simulink model "sgMdl_ModbusTCP_1CLI3SRV"  (R2024b)
settings: Solver=FixedStepAuto  StartTime=0.0  StopTime=inf  RelTol=1e-3  EnableMultiTasking=on
libraries: speedgoatlib_mbtcp x27, slrealtimeutilitieslib x20
Description:
  | Native Modbus TCP Multi-Node Loopback
settings Model: sg_rtwmakecfg_data=_sg_IO75X_v1_2_0__sg_netxLib_MSVC140_  ModifiedByFormat=Speedgoat  SimulationMode=external  ExtModeTrigDuration=100000  Creator=Speedgoat  LastModifiedBy=Speedgoat
settings SolverCC: ConcurrentTasks=on  AlgebraicLoopSolver=TrustRegion  PositivePriorityOrder=on  AutoInsertRateTranBlk=on  InsertRTBMode=Never (minimum delay)
settings DataIOCC: LimitDataPoints=on  SaveFormat=StructureWithTime  ReturnWorkspaceOutputs=off
settings OptimizationCC: BlockReduction=off  BooleanDataType=off  OptimizeBlockIOStorage=off  BufferReuse=off  GlobalBufferReuse=off  ExpressionFolding=off  LocalBlockOutputs=off  OptimizeDataStoreBuffers=off  BusAssignmentInplaceUpdate=off
settings DebuggingCC: SaveWithParameterizedLinksMsg=none  UnderspecifiedInitializationDetection=Classic  MergeDetectMultiDrivingBlocksExec=none  SignalResolutionControl=TryResolveAllWithWarning  InheritedTsInSrcMsg=none  TasksWithSamePriorityMsg=none  ParameterOverflowMsg=warning  UnconnectedInputMsg=warning  UnconnectedOutputMsg=warning  UnconnectedLineMsg=warning  SFUnexpectedBacktrackingDiag=warning  SFNoUnconditionalDefaultTransitionDiag=warning  SFExecutionAtInitializationDiag=none  ArithmeticOperatorsInVariantConditions=warning
settings HardwareCC: ProdBitPerLong=64  ProdLongLongMode=on  ProdHWDeviceType=Intel->x86-64 (Linux 64)  TargetBitPerPointer=64  TargetBitPerSizeT=64  TargetBitPerPtrDiffT=64  TargetLongLongMode=on  TargetIntDivRoundTo=Zero  TargetEndianess=LittleEndian  TargetWordSize=64  TargetHWDeviceType=MATLAB Host
settings ModelReferenceCC: EnableRefExpFcnMdlSchedulingChecks=on  PropagateSignalLabelsOutOfModel=off
settings SFSimCC: SimUseLocalCustomCode=off  CustomCodeUndefinedFunction=UseInterfaceOnly
settings RTWCC: Description=Speedgoat Real-Time Target Machine  SystemTargetFile=speedgoat.tlc  TemplateMakefile=slrealtime_default_tmf  RetainRTWFile=on  RTWUseLocalCustomCode=off  Toolchain=Simulink Real-Time Toolchain  BuildConfiguration=Faster Runs  TargetLang=C++  GPUComputeCapability=3.5  DLArmComputeVersion=19.05
settings CodeAppCC: StateflowObjectComments=on
settings SimulinkRealTimeTargetCC: SubcomponentCodeInterfacePackaging=Reusable function  InstructionSetFMA=off  LogToMDFFile=off  SLRTFileLogMaxRuns=10  UseGCCFastMath=on
settings ConfigComp: CovMetricSettings=dw  CovSaveCumulativeToWorkspaceVar=on  CovSaveSingleToWorkspaceVar=on  CovExternalEMLEnable=off  CovBoundaryAbsTol=1.0e-5

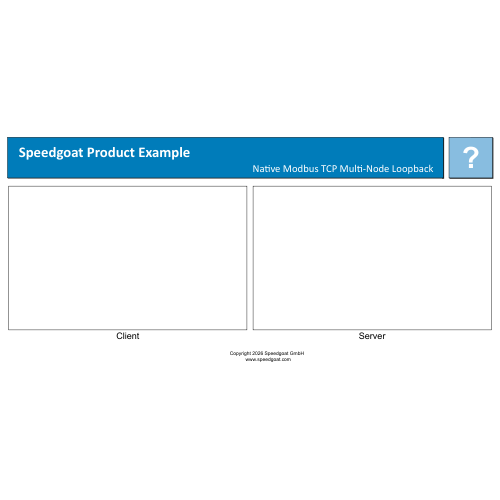
[thumbnail: Simulink's stored preview of the top-level diagram]
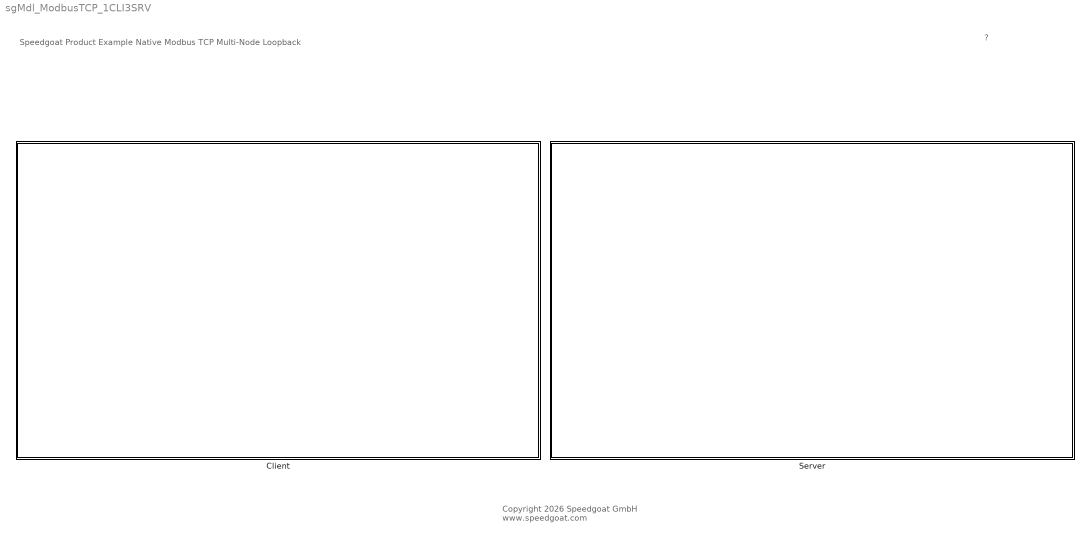
== system sgMdl_ModbusTCP_1CLI3SRV ==
  note: Speedgoat Product Example
      | Native Modbus TCP Multi-Node Loopback
  note: ?
  note: Copyright 2026 Speedgoat GmbH
      |  www.speedgoat.com
  Client : Subsystem
  Server : Subsystem

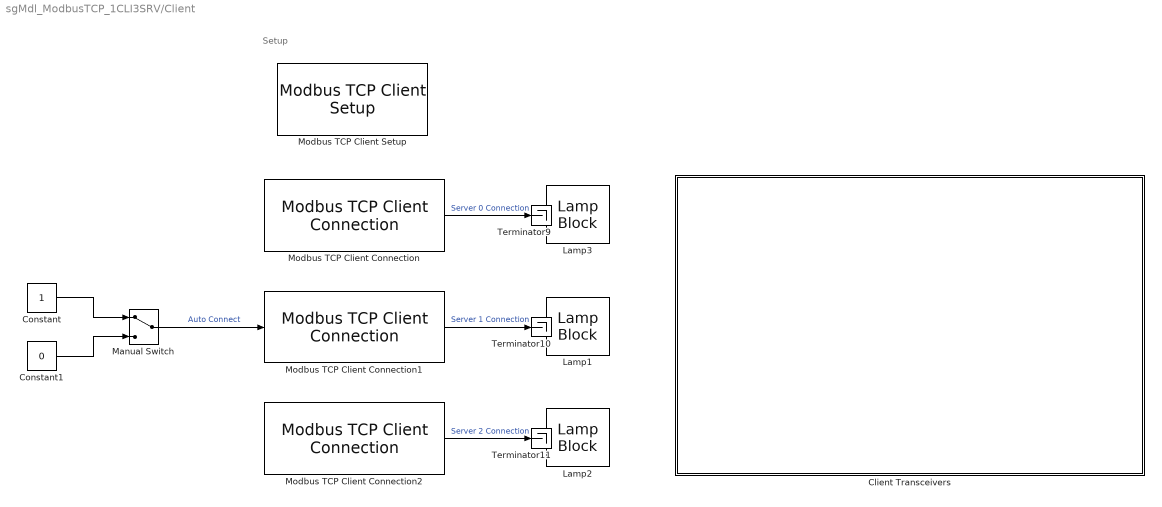
== system sgMdl_ModbusTCP_1CLI3SRV/Client ==
  note: Setup
  Client Transceivers : Subsystem
  Constant : Constant  OutDataTypeStr=boolean
  Constant1 : Constant  Value=0  OutDataTypeStr=boolean
  Lamp1 : LampBlock  LabelPosition=Bottom
  Lamp2 : LampBlock  LabelPosition=Bottom
  Lamp3 : LampBlock  LabelPosition=Bottom
  Manual Switch : ManualSwitch
  Modbus TCP Client Connection : speedgoatlib_mbtcp/Client/Modbus TCP Client Connection  ClientID=10  ConnectionID=0  remoteipAddrStr=IP_Server_00  remoteTCPPort=502  DataSwap=off  parConcurrence=on  AutoConnect=on  SampleTime=-1
      settings: SourceProductName=Simulink Real-Time: Speedgoat I/O Blockset
      settings: AttributesFormatString=|
      | Remote IP: %<remoteipAddrStr>
      | Remote TCP Port: %<remoteTCPPort> | Data Swap: %<DataSwap>
  Modbus TCP Client Connection1 : speedgoatlib_mbtcp/Client/Modbus TCP Client Connection  ClientID=10  ConnectionID=1  remoteipAddrStr=IP_Server_01  remoteTCPPort=502  DataSwap=off  parConcurrence=on  AutoConnect=off  SampleTime=-1
      settings: SourceProductName=Simulink Real-Time: Speedgoat I/O Blockset
      settings: AttributesFormatString=|
      | Remote IP: %<remoteipAddrStr>
      | Remote TCP Port: %<remoteTCPPort> | Data Swap: %<DataSwap>
  Modbus TCP Client Connection2 : speedgoatlib_mbtcp/Client/Modbus TCP Client Connection  ClientID=10  ConnectionID=2  remoteipAddrStr=IP_Server_02  remoteTCPPort=502  DataSwap=off  parConcurrence=on  AutoConnect=on  SampleTime=-1
      settings: SourceProductName=Simulink Real-Time: Speedgoat I/O Blockset
      settings: AttributesFormatString=|
      | Remote IP: %<remoteipAddrStr>
      | Remote TCP Port: %<remoteTCPPort> | Data Swap: %<DataSwap>
  Modbus TCP Client Setup : speedgoatlib_mbtcp/Client/Modbus TCP Client Setup  ClientID=10  IpAddrStr=IP_Client_00  SampleTime=-1
      settings: AttributesFormatString=Local IP: %<IpAddrStr>  SourceProductName=Simulink Real-Time: Speedgoat I/O Blockset
  Terminator10 : Terminator
  Terminator11 : Terminator
  Terminator9 : Terminator
  wires:
  Constant1/1 -> Manual Switch/2
  Constant/1 -> Manual Switch/1
  Modbus TCP Client Connection1/1 -> Terminator10/1  "Server 1 Connection"
  Modbus TCP Client Connection2/1 -> Terminator11/1  "Server 2 Connection"
  Manual Switch/1 -> Modbus TCP Client Connection1/1  "Auto Connect"
  Modbus TCP Client Connection/1 -> Terminator9/1  "Server 0 Connection"

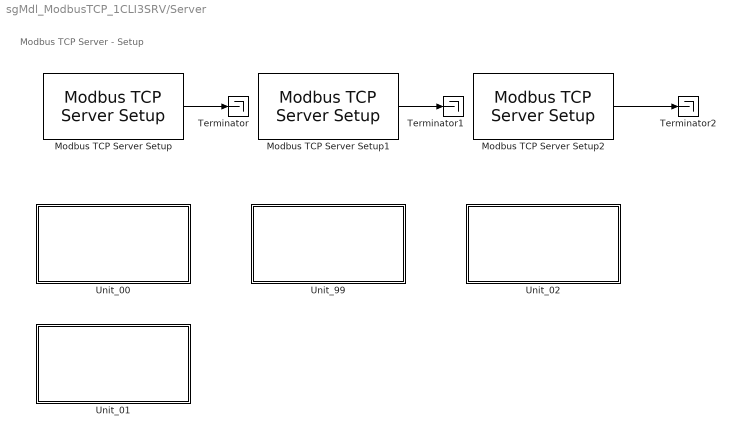
== system sgMdl_ModbusTCP_1CLI3SRV/Server ==
  note: Modbus TCP Server - Setup
  Modbus TCP Server Setup : speedgoatlib_mbtcp/Server/Modbus TCP Server Setup  ServerID=0  IpAddrStr=IP_Server_00  TcpPort=502  Units=[0,1]  TableDim=[10,10,10,10;255,255,255,255]  RespDelay=0  ByteSwap=off  KeepAlive=1  SampleTime=-1
      settings: SourceProductName=Simulink Real-Time: Speedgoat I/O Blockset
      settings: AttributesFormatString=|
      | Local IP: %<IpAddrStr>
      | Local TCP Port: %<TCPPort> | Units: %<Units>
  Modbus TCP Server Setup1 : speedgoatlib_mbtcp/Server/Modbus TCP Server Setup  ServerID=1  IpAddrStr=IP_Server_01  TcpPort=502  Units=[99]  TableDim=[64,64,64,64]  RespDelay=0  ByteSwap=off  KeepAlive=0  SampleTime=-1
      settings: SourceProductName=Simulink Real-Time: Speedgoat I/O Blockset
      settings: AttributesFormatString=|
      | Local IP: %<IpAddrStr>
      | Local TCP Port: %<TCPPort> | Units: %<Units>
  Modbus TCP Server Setup2 : speedgoatlib_mbtcp/Server/Modbus TCP Server Setup  ServerID=2  IpAddrStr=IP_Server_02  TcpPort=502  Units=[2]  TableDim=[64,64,64,64]  RespDelay=0  ByteSwap=off  KeepAlive=0  SampleTime=-1
      settings: SourceProductName=Simulink Real-Time: Speedgoat I/O Blockset
      settings: AttributesFormatString=|
      | Local IP: %<IpAddrStr>
      | Local TCP Port: %<TCPPort> | Units: %<Units>
  Terminator : Terminator
  Terminator1 : Terminator
  Terminator2 : Terminator
  Unit_00 : Subsystem
  Unit_01 : Subsystem
  Unit_02 : Subsystem
  Unit_99 : Subsystem
  wires:
  Modbus TCP Server Setup2/1 -> Terminator2/1
  Modbus TCP Server Setup1/1 -> Terminator1/1
  Modbus TCP Server Setup/1 -> Terminator/1

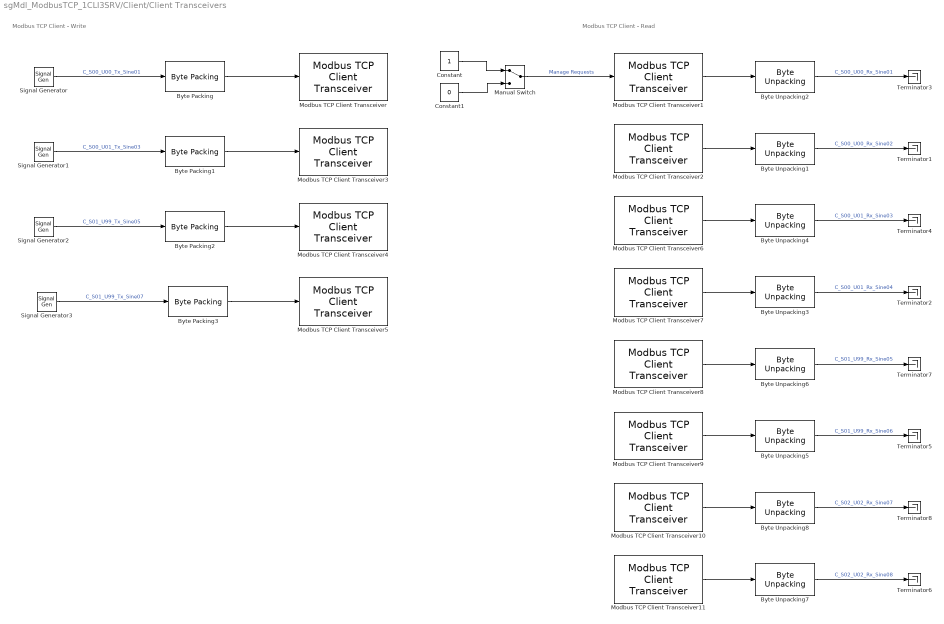
== system sgMdl_ModbusTCP_1CLI3SRV/Client/Client Transceivers ==
  note: Modbus TCP Client - Write
  note: Modbus TCP Client - Read
  Byte Packing{,1..3} (4 alike) : slrealtimeutilitieslib/Byte Packing  MaskPackedDataType=uint16  MaskUnpackedDataTypes={'double'}  MaskAlignment=1
  Byte Unpacking{1..8} (8 alike) : slrealtimeutilitieslib/Byte Unpacking  MaskUnpackedDataTypes={'double'}  MaskUnpackedDataSizes={[1]}  MaskAlignment=1
  Constant : Constant  OutDataTypeStr=boolean
  Constant1 : Constant  Value=0  OutDataTypeStr=boolean
  Manual Switch : ManualSwitch
  Modbus TCP Client Transceiver : speedgoatlib_mbtcp/Client/Modbus TCP Client Transceiver  ClientID=10  ConnectionID=0  remoteUnitID=0  FunctionCode=FC16 (Write Multiple Holding Registers)  DataIndex=0  DataQuantity=4  PollIntervall=50  EnaSend=off  SampleTime=-1  UpdateChange=off
      settings: SourceProductName=Simulink Real-Time: Speedgoat I/O Blockset
      settings: AttributesFormatString=|
      | %<FunctionCode>
      | Server Unit: %<remoteUnitID> | Address Index: %<DataIndex> | Quantity: %<DataQuantity>
  Modbus TCP Client Transceiver1 : speedgoatlib_mbtcp/Client/Modbus TCP Client Transceiver  ClientID=10  ConnectionID=0  remoteUnitID=0  FunctionCode=FC3 (Read Multiple Holding Registers)  DataIndex=0  DataQuantity=4  PollIntervall=50  EnaSend=on  SampleTime=-1  UpdateChange=off
      settings: SourceProductName=Simulink Real-Time: Speedgoat I/O Blockset
      settings: AttributesFormatString=|
      | %<FunctionCode>
      | Server Unit: %<remoteUnitID> | Address Index: %<DataIndex> | Quantity: %<DataQuantity>
  Modbus TCP Client Transceiver10 : speedgoatlib_mbtcp/Client/Modbus TCP Client Transceiver  ClientID=10  ConnectionID=2  remoteUnitID=2  FunctionCode=FC3 (Read Multiple Holding Registers)  DataIndex=0  DataQuantity=4  PollIntervall=50  EnaSend=off  SampleTime=-1  UpdateChange=off
      settings: SourceProductName=Simulink Real-Time: Speedgoat I/O Blockset
      settings: AttributesFormatString=|
      | %<FunctionCode>
      | Server Unit: %<remoteUnitID> | Address Index: %<DataIndex> | Quantity: %<DataQuantity>
  Modbus TCP Client Transceiver11 : speedgoatlib_mbtcp/Client/Modbus TCP Client Transceiver  ClientID=10  ConnectionID=2  remoteUnitID=2  FunctionCode=FC4 (Read Multiple Input Registers)  DataIndex=0  DataQuantity=4  PollIntervall=50  EnaSend=off  SampleTime=-1  UpdateChange=off
      settings: SourceProductName=Simulink Real-Time: Speedgoat I/O Blockset
      settings: AttributesFormatString=|
      | %<FunctionCode>
      | Server Unit: %<remoteUnitID> | Address Index: %<DataIndex> | Quantity: %<DataQuantity>
  Modbus TCP Client Transceiver2 : speedgoatlib_mbtcp/Client/Modbus TCP Client Transceiver  ClientID=10  ConnectionID=0  remoteUnitID=0  FunctionCode=FC4 (Read Multiple Input Registers)  DataIndex=0  DataQuantity=4  PollIntervall=50  EnaSend=off  SampleTime=-1  UpdateChange=off
      settings: SourceProductName=Simulink Real-Time: Speedgoat I/O Blockset
      settings: AttributesFormatString=|
      | %<FunctionCode>
      | Server Unit: %<remoteUnitID> | Address Index: %<DataIndex> | Quantity: %<DataQuantity>
  Modbus TCP Client Transceiver3 : speedgoatlib_mbtcp/Client/Modbus TCP Client Transceiver  ClientID=10  ConnectionID=0  remoteUnitID=1  FunctionCode=FC16 (Write Multiple Holding Registers)  DataIndex=0  DataQuantity=4  PollIntervall=50  EnaSend=off  SampleTime=-1  UpdateChange=off
      settings: SourceProductName=Simulink Real-Time: Speedgoat I/O Blockset
      settings: AttributesFormatString=|
      | %<FunctionCode>
      | Server Unit: %<remoteUnitID> | Address Index: %<DataIndex> | Quantity: %<DataQuantity>
  Modbus TCP Client Transceiver4 : speedgoatlib_mbtcp/Client/Modbus TCP Client Transceiver  ClientID=10  ConnectionID=1  remoteUnitID=99  FunctionCode=FC16 (Write Multiple Holding Registers)  DataIndex=0  DataQuantity=4  PollIntervall=50  EnaSend=off  SampleTime=-1  UpdateChange=off
      settings: SourceProductName=Simulink Real-Time: Speedgoat I/O Blockset
      settings: AttributesFormatString=|
      | %<FunctionCode>
      | Server Unit: %<remoteUnitID> | Address Index: %<DataIndex> | Quantity: %<DataQuantity>
  Modbus TCP Client Transceiver5 : speedgoatlib_mbtcp/Client/Modbus TCP Client Transceiver  ClientID=10  ConnectionID=2  remoteUnitID=2  FunctionCode=FC16 (Write Multiple Holding Registers)  DataIndex=0  DataQuantity=4  PollIntervall=50  EnaSend=off  SampleTime=-1  UpdateChange=off
      settings: SourceProductName=Simulink Real-Time: Speedgoat I/O Blockset
      settings: AttributesFormatString=|
      | %<FunctionCode>
      | Server Unit: %<remoteUnitID> | Address Index: %<DataIndex> | Quantity: %<DataQuantity>
  Modbus TCP Client Transceiver6 : speedgoatlib_mbtcp/Client/Modbus TCP Client Transceiver  ClientID=10  ConnectionID=0  remoteUnitID=1  FunctionCode=FC3 (Read Multiple Holding Registers)  DataIndex=0  DataQuantity=4  PollIntervall=50  EnaSend=off  SampleTime=-1  UpdateChange=off
      settings: SourceProductName=Simulink Real-Time: Speedgoat I/O Blockset
      settings: AttributesFormatString=|
      | %<FunctionCode>
      | Server Unit: %<remoteUnitID> | Address Index: %<DataIndex> | Quantity: %<DataQuantity>
  Modbus TCP Client Transceiver7 : speedgoatlib_mbtcp/Client/Modbus TCP Client Transceiver  ClientID=10  ConnectionID=0  remoteUnitID=1  FunctionCode=FC4 (Read Multiple Input Registers)  DataIndex=0  DataQuantity=4  PollIntervall=50  EnaSend=off  SampleTime=-1  UpdateChange=off
      settings: SourceProductName=Simulink Real-Time: Speedgoat I/O Blockset
      settings: AttributesFormatString=|
      | %<FunctionCode>
      | Server Unit: %<remoteUnitID> | Address Index: %<DataIndex> | Quantity: %<DataQuantity>
  Modbus TCP Client Transceiver8 : speedgoatlib_mbtcp/Client/Modbus TCP Client Transceiver  ClientID=10  ConnectionID=1  remoteUnitID=99  FunctionCode=FC3 (Read Multiple Holding Registers)  DataIndex=0  DataQuantity=4  PollIntervall=50  EnaSend=off  SampleTime=-1  UpdateChange=off
      settings: SourceProductName=Simulink Real-Time: Speedgoat I/O Blockset
      settings: AttributesFormatString=|
      | %<FunctionCode>
      | Server Unit: %<remoteUnitID> | Address Index: %<DataIndex> | Quantity: %<DataQuantity>
  Modbus TCP Client Transceiver9 : speedgoatlib_mbtcp/Client/Modbus TCP Client Transceiver  ClientID=10  ConnectionID=1  remoteUnitID=99  FunctionCode=FC4 (Read Multiple Input Registers)  DataIndex=0  DataQuantity=4  PollIntervall=50  EnaSend=off  SampleTime=-1  UpdateChange=off
      settings: SourceProductName=Simulink Real-Time: Speedgoat I/O Blockset
      settings: AttributesFormatString=|
      | %<FunctionCode>
      | Server Unit: %<remoteUnitID> | Address Index: %<DataIndex> | Quantity: %<DataQuantity>
  Signal Generator : SignalGenerator  Amplitude=10  Frequency=0.1  Units=rad/sec
  Signal Generator1 : SignalGenerator  Amplitude=30  Frequency=0.3  Units=rad/sec
  Signal Generator2 : SignalGenerator  Amplitude=50  Frequency=0.5  Units=rad/sec
  Signal Generator3 : SignalGenerator  Amplitude=70  Frequency=0.7  Units=rad/sec
  Terminator{1..8} (8 alike) : Terminator
  wires:
  Modbus TCP Client Transceiver1/1 -> Byte Unpacking2/1
  Signal Generator/1 -> Byte Packing/1  "C_S00_U00_Tx_Sine01"
  Byte Unpacking1/1 -> Terminator1/1  "C_S00_U00_Rx_Sine02"
  Modbus TCP Client Transceiver2/1 -> Byte Unpacking1/1
  Byte Packing/1 -> Modbus TCP Client Transceiver/1
  Byte Unpacking2/1 -> Terminator3/1  "C_S00_U00_Rx_Sine01"
  Signal Generator1/1 -> Byte Packing1/1  "C_S00_U01_Tx_Sine03"
  Byte Packing1/1 -> Modbus TCP Client Transceiver3/1
  Byte Packing2/1 -> Modbus TCP Client Transceiver4/1
  Signal Generator2/1 -> Byte Packing2/1  "C_S01_U99_Tx_Sine05"
  Signal Generator3/1 -> Byte Packing3/1  "C_S01_U99_Tx_Sine07"
  Byte Packing3/1 -> Modbus TCP Client Transceiver5/1
  Byte Unpacking4/1 -> Terminator4/1  "C_S00_U01_Rx_Sine03"
  Modbus TCP Client Transceiver7/1 -> Byte Unpacking3/1
  Byte Unpacking3/1 -> Terminator2/1  "C_S00_U01_Rx_Sine04"
  Modbus TCP Client Transceiver6/1 -> Byte Unpacking4/1
  Modbus TCP Client Transceiver10/1 -> Byte Unpacking8/1
  Byte Unpacking7/1 -> Terminator6/1  "C_S02_U02_Rx_Sine08"
  Modbus TCP Client Transceiver11/1 -> Byte Unpacking7/1
  Byte Unpacking8/1 -> Terminator8/1  "C_S02_U02_Rx_Sine07"
  Byte Unpacking6/1 -> Terminator7/1  "C_S01_U99_Rx_Sine05"
  Modbus TCP Client Transceiver9/1 -> Byte Unpacking5/1
  Byte Unpacking5/1 -> Terminator5/1  "C_S01_U99_Rx_Sine06"
  Modbus TCP Client Transceiver8/1 -> Byte Unpacking6/1
  Manual Switch/1 -> Modbus TCP Client Transceiver1/1  "Manage Requests"
  Constant1/1 -> Manual Switch/2
  Constant/1 -> Manual Switch/1

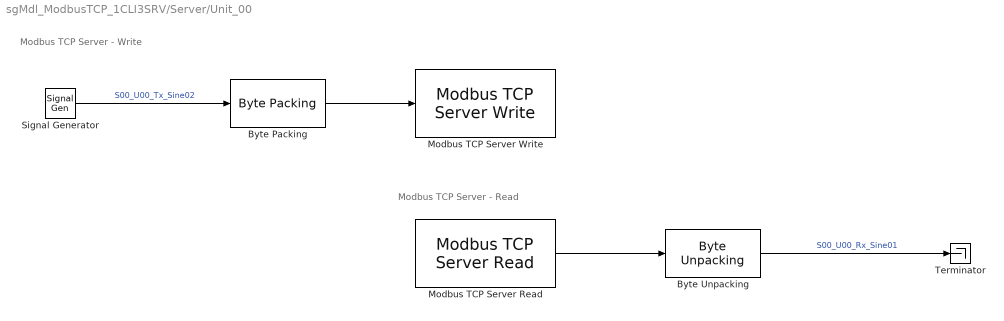
== system sgMdl_ModbusTCP_1CLI3SRV/Server/Unit_00 ==
  note: Modbus TCP Server - Write
  note: Modbus TCP Server - Read
  Byte Packing : slrealtimeutilitieslib/Byte Packing  MaskPackedDataType=uint16  MaskUnpackedDataTypes={'double'}  MaskAlignment=1
  Byte Unpacking : slrealtimeutilitieslib/Byte Unpacking  MaskUnpackedDataTypes={'double'}  MaskUnpackedDataSizes={[1]}  MaskAlignment=1
  Modbus TCP Server Read : speedgoatlib_mbtcp/Server/Modbus TCP Server Read  ServerID=0  UnitID=0  DataTable=Holding Registers  DataIndex=0  DataQuantity=4  SampleTime=-1
      settings: SourceProductName=Simulink Real-Time: Speedgoat I/O Blockset
      settings: AttributesFormatString=|
      | Data Type: %<DataTable>
      | Data Index: %<DataIndex> | Quantity: %<DataQuantity>
  Modbus TCP Server Write : speedgoatlib_mbtcp/Server/Modbus TCP Server Write  ServerID=0  UnitID=0  DataTable=Input Registers  DataIndex=0  DataQuantity=4  SampleTime=-1
      settings: SourceProductName=Simulink Real-Time: Speedgoat I/O Blockset
      settings: AttributesFormatString=|
      | Data Type: %<DataTable>
      | Data Index: %<DataIndex> | Quantity: %<DataQuantity>
  Signal Generator : SignalGenerator  Amplitude=20  Frequency=0.2  Units=rad/sec
  Terminator : Terminator
  wires:
  Modbus TCP Server Read/1 -> Byte Unpacking/1
  Byte Unpacking/1 -> Terminator/1  "S00_U00_Rx_Sine01"
  Byte Packing/1 -> Modbus TCP Server Write/1
  Signal Generator/1 -> Byte Packing/1  "S00_U00_Tx_Sine02"

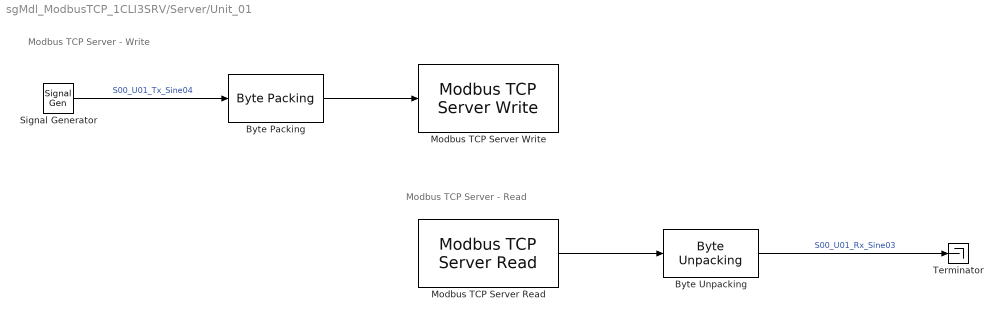
== system sgMdl_ModbusTCP_1CLI3SRV/Server/Unit_01 ==
  note: Modbus TCP Server - Read
  note: Modbus TCP Server - Write
  Byte Packing : slrealtimeutilitieslib/Byte Packing  MaskPackedDataType=uint16  MaskUnpackedDataTypes={'double'}  MaskAlignment=1
  Byte Unpacking : slrealtimeutilitieslib/Byte Unpacking  MaskUnpackedDataTypes={'double'}  MaskUnpackedDataSizes={[1]}  MaskAlignment=1
  Modbus TCP Server Read : speedgoatlib_mbtcp/Server/Modbus TCP Server Read  ServerID=0  UnitID=1  DataTable=Holding Registers  DataIndex=0  DataQuantity=4  SampleTime=-1
      settings: SourceProductName=Simulink Real-Time: Speedgoat I/O Blockset
      settings: AttributesFormatString=|
      | Data Type: %<DataTable>
      | Data Index: %<DataIndex> | Quantity: %<DataQuantity>
  Modbus TCP Server Write : speedgoatlib_mbtcp/Server/Modbus TCP Server Write  ServerID=0  UnitID=1  DataTable=Input Registers  DataIndex=0  DataQuantity=4  SampleTime=-1
      settings: SourceProductName=Simulink Real-Time: Speedgoat I/O Blockset
      settings: AttributesFormatString=|
      | Data Type: %<DataTable>
      | Data Index: %<DataIndex> | Quantity: %<DataQuantity>
  Signal Generator : SignalGenerator  Amplitude=40  Frequency=0.4  Units=rad/sec
  Terminator : Terminator
  wires:
  Signal Generator/1 -> Byte Packing/1  "S00_U01_Tx_Sine04"
  Byte Packing/1 -> Modbus TCP Server Write/1
  Byte Unpacking/1 -> Terminator/1  "S00_U01_Rx_Sine03"
  Modbus TCP Server Read/1 -> Byte Unpacking/1

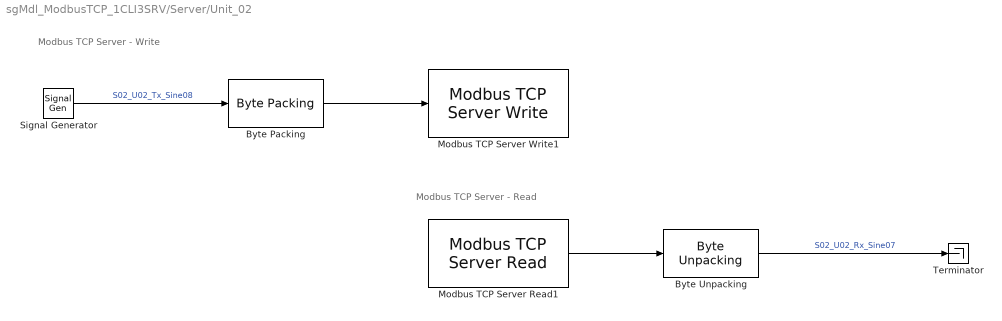
== system sgMdl_ModbusTCP_1CLI3SRV/Server/Unit_02 ==
  note: Modbus TCP Server - Read
  note: Modbus TCP Server - Write
  Byte Packing : slrealtimeutilitieslib/Byte Packing  MaskPackedDataType=uint16  MaskUnpackedDataTypes={'double'}  MaskAlignment=1
  Byte Unpacking : slrealtimeutilitieslib/Byte Unpacking  MaskUnpackedDataTypes={'double'}  MaskUnpackedDataSizes={[1]}  MaskAlignment=1
  Modbus TCP Server Read1 : speedgoatlib_mbtcp/Server/Modbus TCP Server Read  ServerID=2  UnitID=2  DataTable=Holding Registers  DataIndex=0  DataQuantity=4  SampleTime=-1
      settings: SourceProductName=Simulink Real-Time: Speedgoat I/O Blockset
      settings: AttributesFormatString=|
      | Data Type: %<DataTable>
      | Data Index: %<DataIndex> | Quantity: %<DataQuantity>
  Modbus TCP Server Write1 : speedgoatlib_mbtcp/Server/Modbus TCP Server Write  ServerID=2  UnitID=2  DataTable=Input Registers  DataIndex=0  DataQuantity=4  SampleTime=-1
      settings: SourceProductName=Simulink Real-Time: Speedgoat I/O Blockset
      settings: AttributesFormatString=|
      | Data Type: %<DataTable>
      | Data Index: %<DataIndex> | Quantity: %<DataQuantity>
  Signal Generator : SignalGenerator  Amplitude=80  Frequency=0.8  Units=rad/sec
  Terminator : Terminator
  wires:
  Modbus TCP Server Read1/1 -> Byte Unpacking/1
  Byte Unpacking/1 -> Terminator/1  "S02_U02_Rx_Sine07"
  Byte Packing/1 -> Modbus TCP Server Write1/1
  Signal Generator/1 -> Byte Packing/1  "S02_U02_Tx_Sine08"

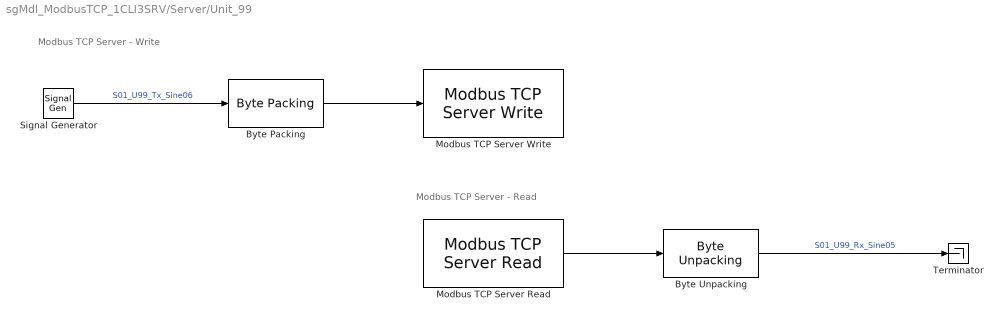
== system sgMdl_ModbusTCP_1CLI3SRV/Server/Unit_99 ==
  note: Modbus TCP Server - Read
  note: Modbus TCP Server - Write
  Byte Packing : slrealtimeutilitieslib/Byte Packing  MaskPackedDataType=uint16  MaskUnpackedDataTypes={'double'}  MaskAlignment=1
  Byte Unpacking : slrealtimeutilitieslib/Byte Unpacking  MaskUnpackedDataTypes={'double'}  MaskUnpackedDataSizes={[1]}  MaskAlignment=1
  Modbus TCP Server Read : speedgoatlib_mbtcp/Server/Modbus TCP Server Read  ServerID=1  UnitID=99  DataTable=Holding Registers  DataIndex=0  DataQuantity=4  SampleTime=-1
      settings: SourceProductName=Simulink Real-Time: Speedgoat I/O Blockset
      settings: AttributesFormatString=|
      | Data Type: %<DataTable>
      | Data Index: %<DataIndex> | Quantity: %<DataQuantity>
  Modbus TCP Server Write : speedgoatlib_mbtcp/Server/Modbus TCP Server Write  ServerID=1  UnitID=99  DataTable=Input Registers  DataIndex=0  DataQuantity=4  SampleTime=-1
      settings: SourceProductName=Simulink Real-Time: Speedgoat I/O Blockset
      settings: AttributesFormatString=|
      | Data Type: %<DataTable>
      | Data Index: %<DataIndex> | Quantity: %<DataQuantity>
  Signal Generator : SignalGenerator  Amplitude=60  Frequency=0.6  Units=rad/sec
  Terminator : Terminator
  wires:
  Signal Generator/1 -> Byte Packing/1  "S01_U99_Tx_Sine06"
  Byte Packing/1 -> Modbus TCP Server Write/1
  Byte Unpacking/1 -> Terminator/1  "S01_U99_Rx_Sine05"
  Modbus TCP Server Read/1 -> Byte Unpacking/1
